simulink model "miniprojekt_rownania_stanu"  (R2022b)
settings: Solver=VariableStepAuto  StartTime=0.0  StopTime=10.0  RelTol=1e-3
values from neighbouring files (symbols this model uses):
  A = [-a1/A1 a1/A1; a1/A2 -(a1+a2)/A2]    [lab8.m]    (also in m.m = [(-(cp*fk*rop)-K1-Kp)/Cvw Kp/Cvw; Kp/Cvp -(Kp+K2)/Cvp]; miniprojekt.m = [(-cpp*rop*Fk0-Ks1-K0)/Cv1, K0/Cv1; (K0+cpp*rop*Fk0)/Cv2 (-K)
  B = [1/A1 0; 0 1/A2]    [lab8.m]    (also in m.m = [K1/Cvw (Cvp*fk*rop)/Cvw; K2/Cvp 0]; miniprojekt.m = [(cpp*rop*Fk0)/Cv1, Ks1/Cv1; 0, Ks2/Cv2])
  C = [1,0;0,1]    [lab8.m]    (also in m.m; miniprojekt.m)
  D = [0,0;0,0]    [lab8.m]    (also in m.m; miniprojekt.m)
  dTkz = 0    [m.m]    (also in miniprojekt.m)
  dTzew = 0    [m.m]    (also in miniprojekt.m = 2)
  T0 = [Twew Tp]    [m.m]
  Tkz = TkzN    (= 35)    [m.m]
  Tzew = -20:5:30    [lab1.m]    (also in m.m = -20; skrypt1.m = -30:5:30)
settings Model: Creator=micha  LastModifiedBy=micha

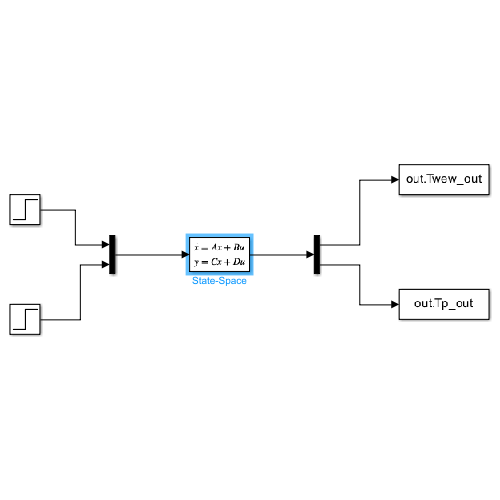
[thumbnail: Simulink's stored preview of the top-level diagram]
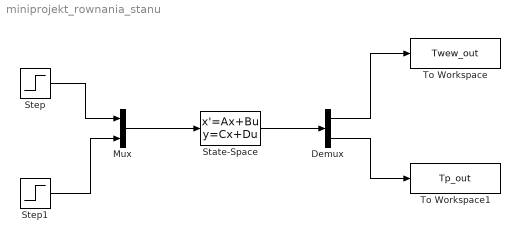
== system miniprojekt_rownania_stanu ==
  Demux : Demux  Outputs=2
  Mux : Mux  Inputs=2
  State-Space : StateSpace  A=A  B=B  C=C  D=D  InitialCondition=T0
  Step : Step  Time=1000  Before=Tzew  After=Tzew+dTzew  SampleTime=0
  Step1 : Step  Time=1000  Before=Tkz  After=Tkz+dTkz  SampleTime=0
  To Workspace : ToWorkspace  VariableName=Twew_out  SampleTime=-1
  To Workspace1 : ToWorkspace  VariableName=Tp_out  SampleTime=-1
  wires:
  State-Space/1 -> Demux/1
  Mux/1 -> State-Space/1
  Demux/1 -> To Workspace/1
  Demux/2 -> To Workspace1/1
  Step/1 -> Mux/1
  Step1/1 -> Mux/2
